simulink model "Problem4"  (R2020a)
settings: Solver=VariableStepAuto  StartTime=0.0  StopTime=10.0  RelTol=1e-3
settings Model: Creator=tnradm  LastModifiedBy=tnradm

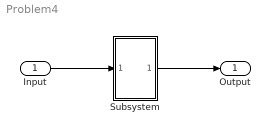
== system Problem4 ==
  Input : Inport  OutDataTypeStr=double  PortDimensions=1  SampleTime=0
  Subsystem : Subsystem  TreatAsAtomicUnit=on
  Output : Outport  OutDataTypeStr=double  PortDimensions=1  SampleTime=0
  wires:
  Input/1 -> Subsystem/1(In1)
  Subsystem/1(Out1) -> Output/1

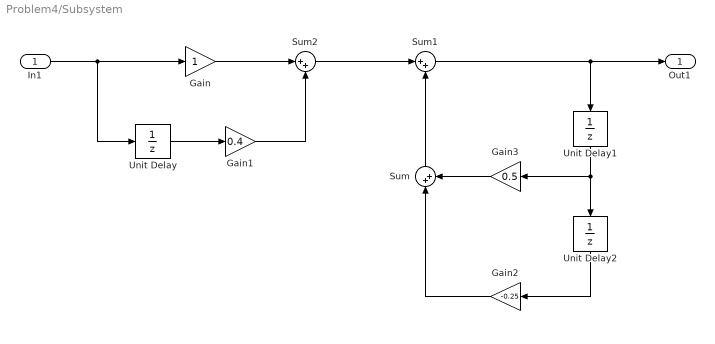
== system Problem4/Subsystem ==
  In1 : Inport
  Gain : Gain
  Gain1 : Gain  Gain=0.4
  Gain2 : Gain  Gain=-0.25
  Gain3 : Gain  Gain=0.5
  Sum : Sum  Inputs=|++
  Sum1 : Sum  Inputs=|++
  Sum2 : Sum  Inputs=|++
  Unit Delay : UnitDelay  SampleTime=-1  HasFrameUpgradeWarning=on
  Unit Delay1 : UnitDelay  SampleTime=-1  HasFrameUpgradeWarning=on
  Unit Delay2 : UnitDelay  SampleTime=-1  HasFrameUpgradeWarning=on
  Out1 : Outport
  wires:
  Gain2/1 -> Sum/1
  Sum/1 -> Sum1/2
  In1/1 -> Gain/1, Unit Delay/1
  Unit Delay2/1 -> Gain2/1
  Gain1/1 -> Sum2/2
  Gain3/1 -> Sum/2
  Unit Delay/1 -> Gain1/1
  Sum1/1 -> Out1/1, Unit Delay1/1
  Gain/1 -> Sum2/1
  Unit Delay1/1 -> Gain3/1, Unit Delay2/1
  Sum2/1 -> Sum1/1
